simulink model "matrixVectTest"  (Simulink 7.8)
settings: Solver=ode45  StartTime=0.0  StopTime=10.0  RelTol=1e-3
settings Model: Creator=benjJohnson  LastModifiedBy=benjJohnson

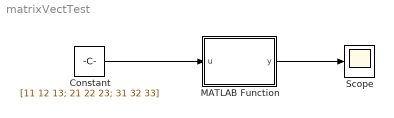
== system matrixVectTest ==
  Constant : Constant  Value=[11 12 13; 21 22 23; 31 32 33]  VectorParams1D=off
  MATLAB Function : MATLAB Function  TreatAsAtomicUnit=on
  Scope : Scope
  wires:
  Constant/1 -> MATLAB Function/1(u)
  MATLAB Function/1(y) -> Scope/1

== matlab function MATLAB Function ==
  data: u input double; y output double
function y = fcn(u)
%#codegen
coder.extrinsic('lower')
y = SpinCalc('DCMtoEA231', 0.01, 0);
